simulink model "LQR_linearized_sim"  (R2025b)
settings: Solver=VariableStepAuto  StartTime=0.0  StopTime=5  RelTol=1e-3
undefined symbols (not defined in the file): A, A_vert, A_xy, B, B_vert, B_xy, bb, C, C_vert, C_xy, D, D_vert, D_xy, dotphi_x_ref, dotphi_y_ref, ic, ic_xy, ic_xz, ic_yz, K, K_vert, K_xy, Kr, N_vert
settings Model: Creator=JPham  LastModifiedBy=JPham

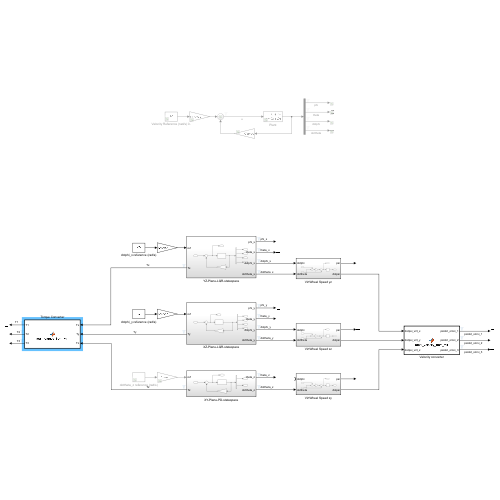
[thumbnail: Simulink's stored preview of the top-level diagram]
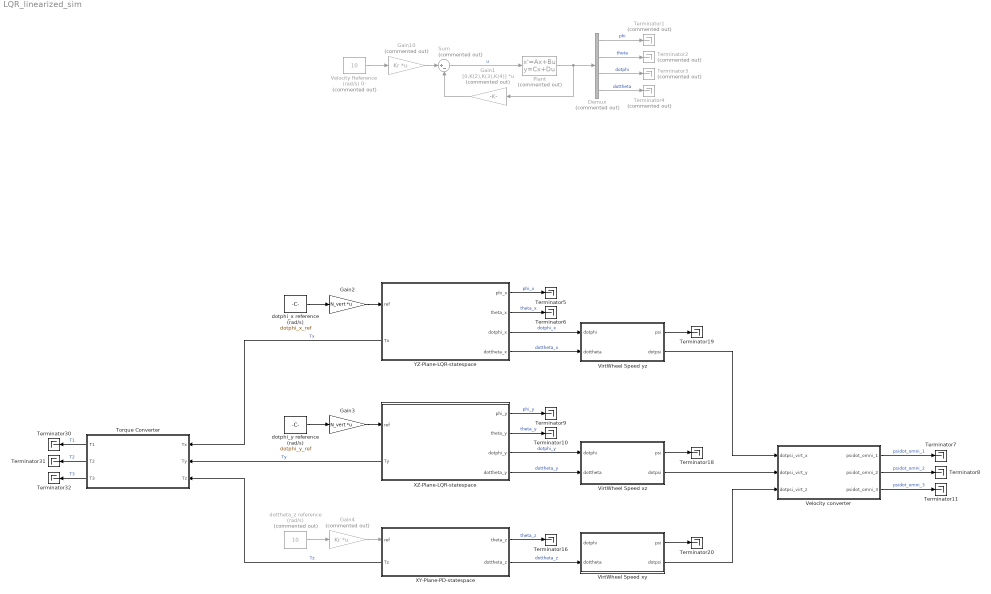
== system LQR_linearized_sim ==
  Demux : Demux  Commented=on
  Gain1 : Gain  Commented=on  Gain=[0,K(2),K(3),K(4)]  Multiplication=Matrix(K*u) (u vector)
  Gain10 : Gain  Commented=on  Gain=Kr  Multiplication=Matrix(K*u) (u vector)
  Gain2 : Gain  Gain=N_vert  Multiplication=Matrix(K*u) (u vector)
  Gain3 : Gain  Gain=N_vert  Multiplication=Matrix(K*u) (u vector)
  Gain4 : Gain  Commented=on  Gain=Kr  Multiplication=Matrix(K*u) (u vector)
  Plant : StateSpace  Commented=on  A=A  B=B  C=C  D=D  InitialCondition=ic  ContinuousStateAttributes={'phi', 'theta', 'dot_phi', 'dot_theta'}
  Sum : Sum  Commented=on  Inputs=|+-
  Terminator{1..4} (4 alike) : Terminator  Commented=on
  Terminator{5..11,16,18..20,30..32} (14 alike) : Terminator
  Torque Converter : MATLAB Function  TreatAsAtomicUnit=on
  Velocity Reference (rad/s) 0- : Constant  Commented=on  Value=10
  Velocity converter : MATLAB Function  TreatAsAtomicUnit=on
  VirtWheel Speed xy : Subsystem
  VirtWheel Speed xz : Subsystem
  VirtWheel Speed yz : Subsystem
  XY-Plane-PD-statespace : Subsystem
      settings: PortSchema="{\"entries\":[{\"content\":{\"sides\":[{\"content\":{\"connectorIds\":[\"In1\",\"Out3\"]},\"type\":\"ConnectorPlacement.EquallySpacedRectSide\",\"uuid\":\"5f48d994-dd0e-425d-b379-0a8fa9f00982\"},{\"content\":{\"connectorIds\":[\"Out1\",\"Out2\"],\"side\":\"RIGHT\"},\"type\":\"ConnectorPlacement.EquallySpacedRectSide\",\"uuid\":\"51765662-8b4a-4d33-9f32-2719c2447504\"},{\"content\":{\"side\":\"TOP\"},\"type\":\"ConnectorPlacement.EquallySpacedRectSide\",\"uuid\":\"80679327-93da-4ce2-be0f-e798abf55726\"}]},\"type\":\"ConnectorPlacement.EquallySpacedConnector\",\"uuid\":\"63065788-10aa-4df6-b18e-3a1aafbfe9ad\"}],\"packageUris\":[\"http://schema.mathworks.com/mf0/Connector/R2020b\"],\"version\":\"1.0\"}"
  XZ-Plane-LQR-statespace : Subsystem
      settings: PortSchema="{\"entries\":[{\"content\":{\"sides\":[{\"content\":{\"connectorIds\":[\"In1\",\"Out5\"]},\"type\":\"ConnectorPlacement.EquallySpacedRectSide\",\"uuid\":\"bad12bff-e47a-4640-8e93-cd5e90d0632f\"},{\"content\":{\"connectorIds\":[\"Out1\",\"Out2\",\"Out3\",\"Out4\"],\"side\":\"RIGHT\"},\"type\":\"ConnectorPlacement.EquallySpacedRectSide\",\"uuid\":\"51ce8fa9-9040-4f84-870e-6aa53e6e757d\"},{\"content\":{\"side\":\"TOP\"},\"type\":\"ConnectorPlacement.EquallySpacedRectSide\",\"uuid\":\"9f672580-11ba-4792-921f-2ef4544f6151\"}]},\"type\":\"ConnectorPlacement.EquallySpacedConnector\",\"uuid\":\"89e14e63-9cf3-48e8-a6f7-9e3aa12bac2b\"}],\"packageUris\":[\"http://schema.mathworks.com/mf0/Connector/R2020b\"],\"version\":\"1.0\"}"
  YZ-Plane-LQR-statespace : Subsystem
      settings: PortSchema="{\"entries\":[{\"content\":{\"sides\":[{\"content\":{\"connectorIds\":[\"In1\",\"Out5\"]},\"type\":\"ConnectorPlacement.EquallySpacedRectSide\",\"uuid\":\"bad12bff-e47a-4640-8e93-cd5e90d0632f\"},{\"content\":{\"connectorIds\":[\"Out1\",\"Out2\",\"Out3\",\"Out4\"],\"side\":\"RIGHT\"},\"type\":\"ConnectorPlacement.EquallySpacedRectSide\",\"uuid\":\"51ce8fa9-9040-4f84-870e-6aa53e6e757d\"},{\"content\":{\"side\":\"TOP\"},\"type\":\"ConnectorPlacement.EquallySpacedRectSide\",\"uuid\":\"9f672580-11ba-4792-921f-2ef4544f6151\"}]},\"type\":\"ConnectorPlacement.EquallySpacedConnector\",\"uuid\":\"89e14e63-9cf3-48e8-a6f7-9e3aa12bac2b\"}],\"packageUris\":[\"http://schema.mathworks.com/mf0/Connector/R2020b\"],\"version\":\"1.0\"}"
  dotphi_x reference (rad/s) : Constant  Value=dotphi_x_ref
  dotphi_y reference (rad/s) : Constant  Value=dotphi_y_ref
  dottheta_z reference (rad/s) : Constant  Commented=on  Value=10
  wires:
  Demux/3 -> Terminator3/1  "dotphi"
  Velocity Reference (rad/s) 0-/1 -> Gain10/1
  Demux/2 -> Terminator2/1  "theta"
  Gain10/1 -> Sum/1
  Demux/1 -> Terminator1/1  "phi"
  Sum/1 -> Plant/1  "u"
  Demux/4 -> Terminator4/1  "dottheta"
  Gain1/1 -> Sum/2
  Plant/1 -> Gain1/1, Demux/1
  YZ-Plane-LQR-statespace/1(phi_x) -> Terminator5/1  "phi_x"
  YZ-Plane-LQR-statespace/2(theta_x) -> Terminator6/1  "theta_x"
  YZ-Plane-LQR-statespace/4(dottheta_x) -> VirtWheel Speed yz/2(dottheta)  "dottheta_x"
  YZ-Plane-LQR-statespace/3(dotphi_x) -> VirtWheel Speed yz/1(dotphi)  "dotphi_x"
  XY-Plane-PD-statespace/2(dottheta_z) -> VirtWheel Speed xy/2(dottheta)  "dottheta_z"
  XY-Plane-PD-statespace/1(theta_z) -> Terminator16/1  "theta_z"
  YZ-Plane-LQR-statespace/5(Tx) -> Torque Converter/1(Tx)  "Tx"
  XZ-Plane-LQR-statespace/5(Ty) -> Torque Converter/2(Ty)  "Ty"
  XY-Plane-PD-statespace/3(Tz) -> Torque Converter/3(Tz)  "Tz"
  VirtWheel Speed yz/1(psi) -> Terminator19/1
  VirtWheel Speed xz/2(dotpsi) -> Velocity converter/2(dotpsi_virt_y)
  VirtWheel Speed xy/2(dotpsi) -> Velocity converter/3(dotpsi_virt_z)
  VirtWheel Speed xz/1(psi) -> Terminator18/1
  VirtWheel Speed xy/1(psi) -> Terminator20/1
  VirtWheel Speed yz/2(dotpsi) -> Velocity converter/1(dotpsi_virt_x)
  Velocity converter/1(psidot_omni_1) -> Terminator7/1  "psidot_omni_1"
  Velocity converter/2(psidot_omni_2) -> Terminator8/1  "psidot_omni_2"
  Velocity converter/3(psidot_omni_3) -> Terminator11/1  "psidot_omni_3"
  Torque Converter/1(T1) -> Terminator30/1  "T1"
  Torque Converter/2(T2) -> Terminator31/1  "T2"
  Torque Converter/3(T3) -> Terminator32/1  "T3"
  XZ-Plane-LQR-statespace/3(dotphi_y) -> VirtWheel Speed xz/1(dotphi)  "dotphi_y"
  XZ-Plane-LQR-statespace/4(dottheta_y) -> VirtWheel Speed xz/2(dottheta)  "dottheta_y"
  XZ-Plane-LQR-statespace/2(theta_y) -> Terminator10/1  "theta_y"
  XZ-Plane-LQR-statespace/1(phi_y) -> Terminator9/1  "phi_y"
  dotphi_x reference (rad/s)/1 -> Gain2/1
  dotphi_y reference (rad/s)/1 -> Gain3/1
  dottheta_z reference (rad/s)/1 -> Gain4/1
  Gain4/1 -> XY-Plane-PD-statespace/1(ref)
  Gain3/1 -> XZ-Plane-LQR-statespace/1(ref)
  Gain2/1 -> YZ-Plane-LQR-statespace/1(ref)

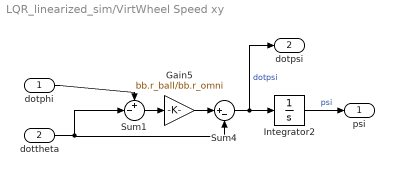
== system LQR_linearized_sim/VirtWheel Speed xy ==
  dotphi : Inport
  dottheta : Inport  Port=2
  Gain5 : Gain  Gain=bb.r_ball/bb.r_omni
  Integrator2 : Integrator
  Sum1 : Sum  Inputs=+-|
  Sum4 : Sum  Inputs=|+-
  psi : Outport
  dotpsi : Outport  Port=2
  wires:
  Sum1/1 -> Gain5/1
  dotphi/1 -> Sum1/1
  Integrator2/1 -> psi/1  "psi"
  Sum4/1 -> Integrator2/1, dotpsi/1  "dotpsi"
  dottheta/1 -> Sum4/2, Sum1/2
  Gain5/1 -> Sum4/1

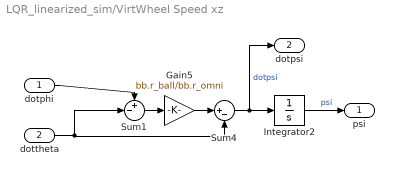
== system LQR_linearized_sim/VirtWheel Speed xz ==
  dotphi : Inport
  dottheta : Inport  Port=2
  Gain5 : Gain  Gain=bb.r_ball/bb.r_omni
  Integrator2 : Integrator
  Sum1 : Sum  Inputs=+-|
  Sum4 : Sum  Inputs=|+-
  psi : Outport
  dotpsi : Outport  Port=2
  wires:
  Gain5/1 -> Sum4/1
  dottheta/1 -> Sum1/2, Sum4/2
  Sum4/1 -> dotpsi/1, Integrator2/1  "dotpsi"
  Integrator2/1 -> psi/1  "psi"
  dotphi/1 -> Sum1/1
  Sum1/1 -> Gain5/1

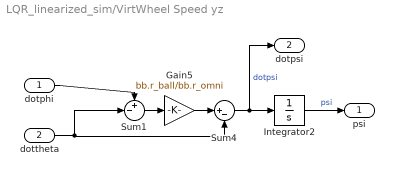
== system LQR_linearized_sim/VirtWheel Speed yz ==
  dotphi : Inport
  dottheta : Inport  Port=2
  Gain5 : Gain  Gain=bb.r_ball/bb.r_omni
  Integrator2 : Integrator
  Sum1 : Sum  Inputs=+-|
  Sum4 : Sum  Inputs=|+-
  psi : Outport
  dotpsi : Outport  Port=2
  wires:
  Sum1/1 -> Gain5/1
  dotphi/1 -> Sum1/1
  Integrator2/1 -> psi/1  "psi"
  Sum4/1 -> Integrator2/1, dotpsi/1  "dotpsi"
  dottheta/1 -> Sum4/2, Sum1/2
  Gain5/1 -> Sum4/1

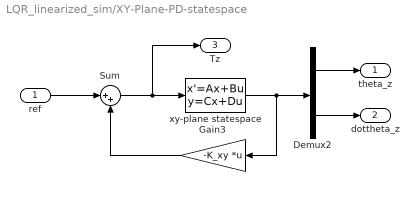
== system LQR_linearized_sim/XY-Plane-PD-statespace ==
  ref : Inport
  Demux2 : Demux  Outputs=2
  Gain3 : Gain  Gain=-K_xy  Multiplication=Matrix(K*u) (u vector)
  Sum : Sum  Inputs=|++
  xy-plane statespace : StateSpace  A=A_xy  B=B_xy  C=C_xy  D=D_xy  InitialCondition=ic_xy  ContinuousStateAttributes={'theta', 'dot_theta'}
  theta_z : Outport
  dottheta_z : Outport  Port=2
  Tz : Outport  Port=3
  wires:
  Demux2/2 -> dottheta_z/1
  xy-plane statespace/1 -> Demux2/1, Gain3/1
  Demux2/1 -> theta_z/1
  Gain3/1 -> Sum/2
  ref/1 -> Sum/1
  Sum/1 -> xy-plane statespace/1, Tz/1

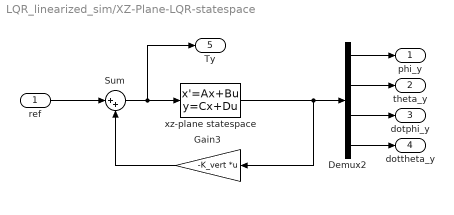
== system LQR_linearized_sim/XZ-Plane-LQR-statespace ==
  ref : Inport
  Demux2 : Demux
  Gain3 : Gain  Gain=-K_vert  Multiplication=Matrix(K*u) (u vector)
  Sum : Sum  Inputs=|++
  xz-plane statespace : StateSpace  A=A_vert  B=B_vert  C=C_vert  D=D_vert  InitialCondition=ic_xz  ContinuousStateAttributes={'phi', 'theta', 'dot_phi', 'dot_theta'}
  phi_y : Outport
  theta_y : Outport  Port=2
  dotphi_y : Outport  Port=3
  dottheta_y : Outport  Port=4
  Ty : Outport  Port=5
  wires:
  Sum/1 -> xz-plane statespace/1, Ty/1
  ref/1 -> Sum/1
  Demux2/1 -> phi_y/1
  Gain3/1 -> Sum/2
  Demux2/3 -> dotphi_y/1
  Demux2/2 -> theta_y/1
  xz-plane statespace/1 -> Demux2/1, Gain3/1
  Demux2/4 -> dottheta_y/1

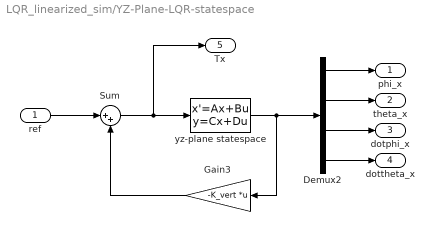
== system LQR_linearized_sim/YZ-Plane-LQR-statespace ==
  ref : Inport
  Demux2 : Demux
  Gain3 : Gain  Gain=-K_vert  Multiplication=Matrix(K*u) (u vector)
  Sum : Sum  Inputs=|++
  yz-plane statespace : StateSpace  A=A_vert  B=B_vert  C=C_vert  D=D_vert  InitialCondition=ic_yz  ContinuousStateAttributes={'phi', 'theta', 'dot_phi', 'dot_theta'}
  phi_x : Outport
  theta_x : Outport  Port=2
  dotphi_x : Outport  Port=3
  dottheta_x : Outport  Port=4
  Tx : Outport  Port=5
  wires:
  Demux2/4 -> dottheta_x/1
  yz-plane statespace/1 -> Gain3/1, Demux2/1
  Demux2/2 -> theta_x/1
  Demux2/3 -> dotphi_x/1
  Gain3/1 -> Sum/2
  Demux2/1 -> phi_x/1
  ref/1 -> Sum/1
  Sum/1 -> Tx/1, yz-plane statespace/1

== matlab function LQR_linearized_sim/Torque Converter ==
  data: Tx input; Ty input; T1 output; Tz input; T2 output; T3 output
function [T1, T2, T3] = real_torques_from_virt(Tx, Ty, Tz)
alpha = params().alpha;
beta  = params().beta;

cosa = cos(alpha);
cb = cos(beta);
sb = sin(beta);

T1 = (1/3) * ( ...
      Tz + (2/cosa) * (Tx*cb - Ty*sb) );

T2 = (1/3) * ( ...
      Tz + (1/cosa) * ( sb*(-sqrt(3)*Tx + Ty) ...
                      - cb*( Tx + sqrt(3)*Ty ) ) );

T3 = (1/3) * ( ...
      Tz + (1/cosa) * ( sb*( sqrt(3)*Tx + Ty) ...
                      + cb*(-Tx + sqrt(3)*Ty ) ) );

end

== matlab function LQR_linearized_sim/Velocity converter ==
  data: dotpsi_virt_x input; dotpsi_virt_y input; psidot_omni_1 output; dotpsi_virt_z input; psidot_omni_2 output; psidot_omni_3 output
% This function convert the velocity of the virtual wheels
% from three planes to the velocity of the omniwheels.
% for beta = 0

function [psidot_omni_1, psidot_omni_2, psidot_omni_3] = ...
    omni_velocity_from_virt(dotpsi_virt_x, dotpsi_virt_y, dotpsi_virt_z)
bb = params();
rads_to_rpm = 30/pi;

psidot_omni_1 = (dotpsi_virt_x * cos(bb.alpha) ...
    + dotpsi_virt_z*sin(bb.alpha))*rads_to_rpm;
psidot_omni_2 = (-0.5 * dotpsi_virt_x * cos(bb.alpha) ...
    - sqrt(3)*dotpsi_virt_y*cos(bb.alpha)/2 ...
    + dotpsi_virt_z*sin(bb.alpha))* rads_to_rpm;
psidot_omni_3 = (-0.5 * dotpsi_virt_x * cos(bb.alpha) ...
    + sqrt(3)*dotpsi_virt_y*cos(bb.alpha)/2 ...
    + dotpsi_virt_z*sin(bb.alpha))* rads_to_rpm;
end
